simulink library "csu_ewp_evaluate_wp_lib"  (R2014b)
settings: Solver=ode45  StartTime=0.0  StopTime=10.0  RelTol=1e-3
libraries: util_info_lib x1
settings Model: Creator=escrane  LastModifiedBy=mstewart

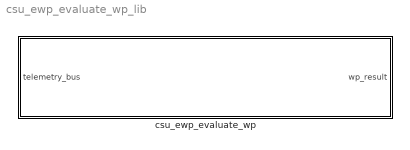
== system csu_ewp_evaluate_wp_lib ==
  csu_ewp_evaluate_wp : Subsystem  mask{wp_id=1, signal_name=est_bus_msg.pos, signal_index=1, comparison_value=0, comparison_type=<=, bitmask_value=0}
      mask prompts: wp_id "Watch Point ID Number"; signal_name "Signal Name"; signal_index "Signal Index"; comparison_value "Comparison Value for WP"; comparison_type "Relational Operator:"; bitmask_value "Bitmask Value for comparison (0 for none)"
      mask init:
      | csu_ewp_evaluate_wp_callback(gcb, signal_name, signal_index, comparison_type, bitmask_value);
      mask TypeOptions comparison_type: == | ~= | < | <= | >= | >
      mask Display:
      | disp(['{\bfWP #' wp_id '}'], 'texmode', 'on');
      | 
      | if bitmask_value == 0
      |     bitmask_str = ' ';
      | else
      |     bitmask_str = [' & 0x' dec2hex(bitmask_value) ' '];
      | end
      | 
      | index_str = ['(' strrep(int2str(signal_index), ' ', ',') ')'];
      | 
      | % Get the un-evaluated string representation of our limit
      | mask_values = get_param(gcb, 'MaskValues');
      | limit_value_string = mask_values{4};
      | 
      | if ~isempty(regexpi(limit_value_string, 'enum_\w+\.'))
      |     limit_value_tokens = regexpi(limit_value_string, 'enum_\w+\.(\w+)', 'tokens', 'once');
      |     limit_value_string = regexprep(upper(limit_value_tokens{1}), '_', '\\_');
      | end
      | 
      | disp(['{\newline\bf' regexprep(signal_name, '_', '\\_') index_str bitmask_str comparison_type ' ' limit_value_string '}'], 'texmode', 'on');
      | % ' }'], 'texmode', 'on')

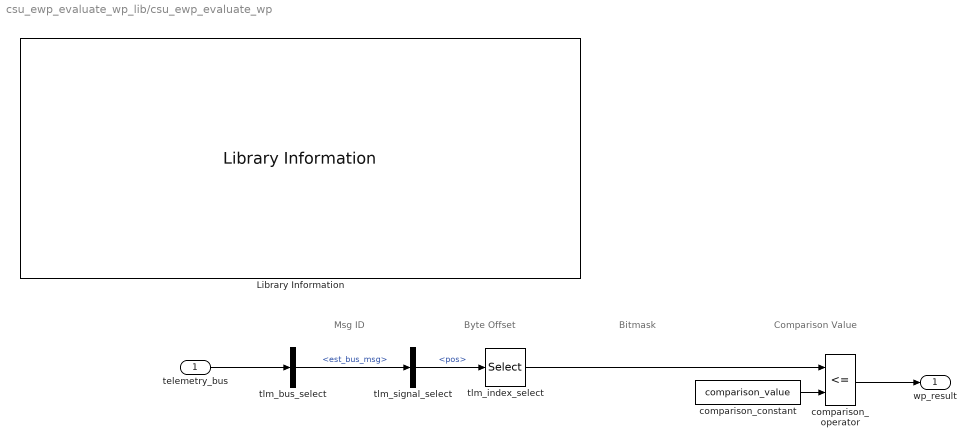
== system csu_ewp_evaluate_wp_lib/csu_ewp_evaluate_wp ==
  note: Msg ID
  note: Byte Offset
  note: Bitmask
  note: Comparison Value
  telemetry_bus : Inport
  Library Information : util_info_lib/Library Information  owner='NONE'
  comparison_constant : Constant  Value=comparison_value  OutDataTypeStr=Inherit: Inherit via back propagation
  comparison_operator : RelationalOperator  Operator=<=  OutDataTypeStr=boolean  InputSameDT=on
  tlm_bus_select : BusSelector  OutputSignals=est_bus_msg
  tlm_index_select : Selector
  tlm_signal_select : BusSelector  OutputSignals=pos
  wp_result : Outport
  wires:
  comparison_operator/1 -> wp_result/1
  telemetry_bus/1 -> tlm_bus_select/1
  tlm_signal_select/1 -> tlm_index_select/1  "<pos>"
  comparison_constant/1 -> comparison_operator/2
  tlm_bus_select/1 -> tlm_signal_select/1  "<est_bus_msg>"
  tlm_index_select/1 -> comparison_operator/1
